simulink model "Exp2_ControlSystemDemo"  (R2017b)
settings: Solver=ode4  StartTime=0.0  StopTime=2000  FixedStep=0.001  RelTol=1e-3
InitFcn:
  | Init_control;
values from neighbouring files (symbols this model uses):
  KiPitchAttitude = 0.0552303199591522 / kFactor    (= 0.0460252666326)    [Init_control.m]
  KiPitchRate = 0.460338699849681 / kFactor    (= 0.383615583208)    [Init_control.m]
  KiRollAttitude = 0.0552303199591522 / kFactor    (= 0.0460252666326)    [Init_control.m]
  KiRollRate = 0.460338699849681 / kFactor    (= 0.383615583208)    [Init_control.m]
  KiYawRate = 0.460338699849681 / kFactor    (= 0.383615583208)    [Init_control.m]
  KpPitchAttitude = 0.630138625117681 / kFactor    (= 0.525115520931)    [Init_control.m]
  KpPitchRate = 1.31533836563383 / kFactor    (= 1.09611530469)    [Init_control.m]
  KpRollAttitude = 0.630138625117681 / kFactor    (= 0.525115520931)    [Init_control.m]
  KpRollRate = 1.31533836563383 / kFactor    (= 1.09611530469)    [Init_control.m]
  KpYawRate = 1.31533836563383 / kFactor    (= 1.09611530469)    [Init_control.m]
undefined symbols (not defined in the file or in its folder): earthRadius, ModelInit_RPM, ModelParam_envAltitude, ModelParam_GlobalNoiseGainSwitch, ModelParam_GPSLatLong, ModelParam_motorCr, ModelParam_motorJm, ModelParam_motorMinThr, ModelParam_motorT, ModelParam_motorWb, ModelParam_rotorCm, ModelParam_rotorCt, ModelParam_uavCCm, ModelParam_uavCd, ModelParam_uavDearo, ModelParam_uavJ, ModelParam_uavMass, ModelParam_uavR, ModelParam_uavType, Receive, Send
libraries: simulink x6, aerolibfltsims x4, aerolib6dof2 x1, aerolibanimutils x1
(part 1 of 2)
settings Model: SimulationMode=accelerator  Creator=dream  LastModifiedBy=dream
settings DebuggingCC: BusObjectLabelMismatch=error
settings CodeAppCC: StateflowObjectComments=on

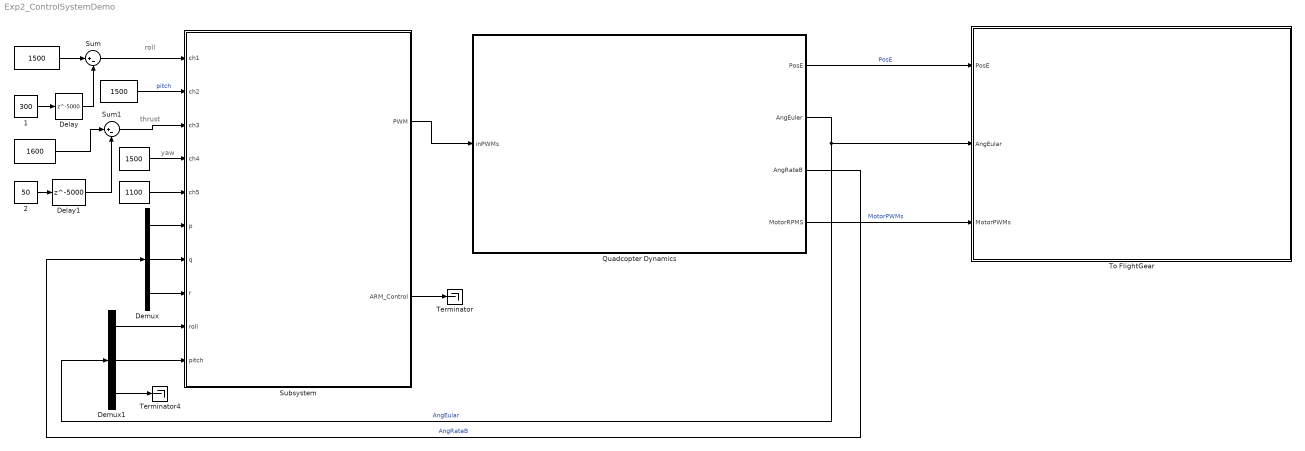
== system Exp2_ControlSystemDemo ==
  note: thrust
  note: yaw
  note: roll
  " " : Constant  Value=1100  OutDataTypeStr=uint16
  "  " : Constant  Value=1500  OutDataTypeStr=uint16
  "   " : Constant  Value=1500  OutDataTypeStr=uint16
  "      " : Constant  Value=1600  OutDataTypeStr=uint16
  "          " : Constant  Value=1500  OutDataTypeStr=uint16
  "  1" : Constant  Value=300  OutDataTypeStr=uint16
  "  2" : Constant  Value=50  OutDataTypeStr=uint16
  Delay : Delay  DelayLength=5000  InitialCondition=0
  Delay1 : Delay  DelayLength=5000  InitialCondition=0
  Demux : Demux  Outputs=3
  Demux1 : Demux  Outputs=3
  Quadcopter Dynamics : Subsystem
      mask Display: image('./icon/F450.png');
  Subsystem : Subsystem
      mask Display: image('./icon/pixhawk.png');
  Sum : Sum  Inputs=|+-
  Sum1 : Sum  Inputs=|+-
  Terminator : Terminator
  Terminator4 : Terminator
  To FlightGear : Subsystem
      mask Display: image('./icon/FlightGear.png');
  wires:
  Quadcopter Dynamics/1(PosE) -> To FlightGear/1(PosE)  "PosE"
  Quadcopter Dynamics/2(AngEuler) -> Demux1/1, To FlightGear/2(AngEular)  "AngEular"
  "   "/1 -> Subsystem/2(ch2)  "pitch"
  "          "/1 -> Subsystem/4(ch4)
  "      "/1 -> Sum1/1
  Quadcopter Dynamics/3(AngRateB) -> Demux/1  "AngRateB"
  " "/1 -> Subsystem/5(ch5)
  Demux/1 -> Subsystem/6(p)
  Demux/2 -> Subsystem/7(q)
  Demux/3 -> Subsystem/8(r)
  Demux1/1 -> Subsystem/9(roll)
  Demux1/2 -> Subsystem/10(pitch)
  Demux1/3 -> Terminator4/1
  "  "/1 -> Sum/1
  Sum/1 -> Subsystem/1(ch1)
  "  1"/1 -> Delay/1
  Delay/1 -> Sum/2
  Quadcopter Dynamics/4(MotorRPMS) -> To FlightGear/3(MotorPWMs)  "MotorPWMs"
  Sum1/1 -> Subsystem/3(ch3)
  "  2"/1 -> Delay1/1
  Delay1/1 -> Sum1/2
  Subsystem/1(PWM) -> Quadcopter Dynamics/1(inPWMs)
  Subsystem/2(ARM_Control) -> Terminator/1

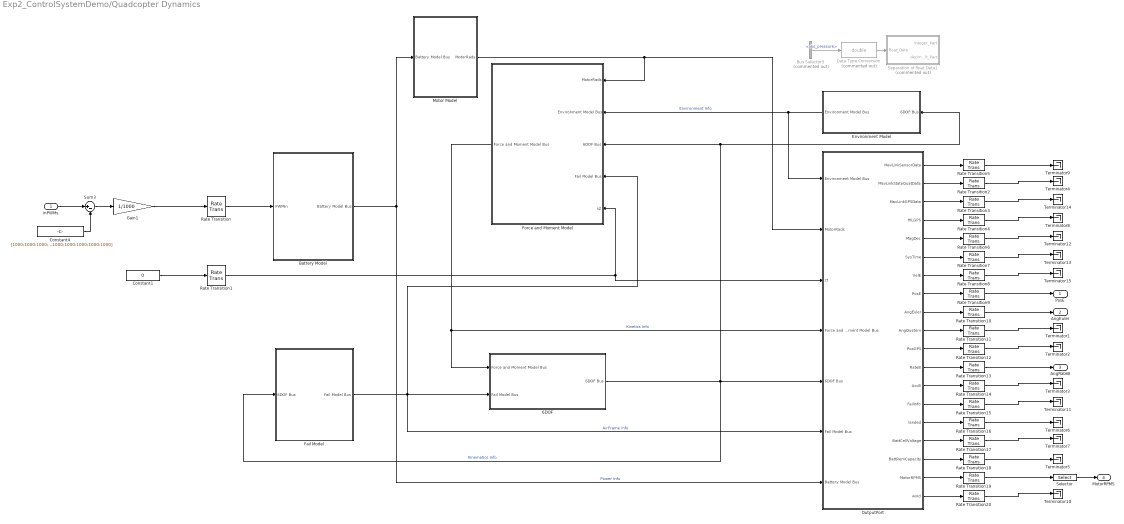
== system Exp2_ControlSystemDemo/Quadcopter Dynamics ==
  inPWMs : Inport  PortDimensions=8
  6DOF : Subsystem
  Battery Model : Subsystem
      mask help: Simulink:masks:GenSFuncDesc_MD
      mask Help: eval('feval(''rtwprivate'',''rtwhelpview'',''rtw_sfcn_block'')');
  Bus Selector3 : BusSelector  Commented=on  OutputSignals=abs_pressure
  Constant1 : Constant  Value=0
  Constant4 : Constant  Value=[1000;1000;1000;1000;1000;1000;1000;1000]
  Data Type Conversion : DataTypeConversion  Commented=on  OutDataTypeStr=double
  Environment Model : Subsystem  mask{sfcnParam1=ModelParam_GPSLatLong, sfcnParam2=ModelParam_GlobalNoiseGainSwitch, sfcnParam3=ModelParam_envAltitude}
      mask prompts: sfcnParam1 "ModelParam_GPSLatLong:"; sfcnParam2 "ModelParam_GlobalNoiseGainSwitch:"; sfcnParam3 "ModelParam_envAltitude:"
      mask help: Simulink:masks:GenSFuncDesc_MD
      mask Help: eval('feval(''rtwprivate'',''rtwhelpview'',''rtw_sfcn_block'')');
  Fail Model : Subsystem  mask{sfcnParam1=ModelParam_uavJ, sfcnParam2=ModelParam_uavMass, sfcnParam3=ModelParam_uavR}
      mask prompts: sfcnParam1 "ModelParam_uavJ:"; sfcnParam2 "ModelParam_uavMass:"; sfcnParam3 "ModelParam_uavR:"
      mask help: Simulink:masks:GenSFuncDesc_MD
      mask Help: eval('feval(''rtwprivate'',''rtwhelpview'',''rtw_sfcn_block'')');
  Force and Moment Model : Subsystem  mask{sfcnParam1=ModelParam_motorJm, sfcnParam2=ModelParam_rotorCm, sfcnParam3=ModelParam_rotorCt, sfcnParam4=ModelParam_uavCCm, sfcnParam5=ModelParam_uavCd, sfcnParam6=ModelParam_uavDearo, sfcnParam7=ModelParam_uavR, sfcnParam8=ModelParam_uavType}
      mask prompts: sfcnParam1 "ModelParam_motorJm:"; sfcnParam2 "ModelParam_rotorCm:"; sfcnParam3 "ModelParam_rotorCt:"; sfcnParam4 "ModelParam_uavCCm:"; sfcnParam5 "ModelParam_uavCd:"; sfcnParam6 "ModelParam_uavDearo:"; sfcnParam7 "ModelParam_uavR:"; sfcnParam8 "ModelParam_uavType:"
      mask help: Simulink:masks:GenSFuncDesc_MD
      mask Help: eval('feval(''rtwprivate'',''rtwhelpview'',''rtw_sfcn_block'')');
  Gain1 : Gain  Gain=1/1000
  Motor Model : Subsystem  mask{sfcnParam1=ModelInit_RPM, sfcnParam2=ModelParam_motorCr, sfcnParam3=ModelParam_motorMinThr, sfcnParam4=ModelParam_motorT, sfcnParam5=ModelParam_motorWb}
      mask prompts: sfcnParam1 "ModelInit_RPM:"; sfcnParam2 "ModelParam_motorCr:"; sfcnParam3 "ModelParam_motorMinThr:"; sfcnParam4 "ModelParam_motorT:"; sfcnParam5 "ModelParam_motorWb:"
      mask help: Simulink:masks:GenSFuncDesc_MD
      mask Help: eval('feval(''rtwprivate'',''rtwhelpview'',''rtw_sfcn_block'')');
  OutputPort : Subsystem  mask{sfcnParam1=ModelParam_GPSLatLong, sfcnParam2=ModelParam_GlobalNoiseGainSwitch, sfcnParam3=ModelParam_envAltitude}
      mask prompts: sfcnParam1 "ModelParam_GPSLatLong:"; sfcnParam2 "ModelParam_GlobalNoiseGainSwitch:"; sfcnParam3 "ModelParam_envAltitude:"
      mask help: Simulink:masks:GenSFuncDesc_MD
      mask Help: eval('feval(''rtwprivate'',''rtwhelpview'',''rtw_sfcn_block'')');
  Rate Transition{,1..20} (21 alike) : RateTransition  OutPortSampleTime=ModelParam_BusSampleRate
  Selector : Selector  InputPortWidth=8  IndexOptions=Index vector (dialog)  Indices=[1 2 3 4]  OutputSizes=1
  Separation of float Data1 : Subsystem  Commented=on  mask{IntUint=1}
      mask prompts: IntUint "整数单位"
      mask help: 分离浮点数的整数和小数部分，这样在Labview MIT模块中可以稳定输出精度
  Sum3 : Sum  Inputs=|+-
  Terminator{1..15} (15 alike) : Terminator
  PosE : Outport
  AngEuler : Outport  Port=2
  AngRateB : Outport  Port=3
  MotorRPMS : Outport  Port=4
  wires:
  Selector/1 -> MotorRPMS/1
  Constant4/1 -> Sum3/2
  inPWMs/1 -> Sum3/1
  Constant1/1 -> Rate Transition1/1
  Sum3/1 -> Gain1/1
  Rate Transition5/1 -> Terminator9/1
  Rate Transition2/1 -> Terminator4/1
  Rate Transition3/1 -> Terminator14/1
  Rate Transition4/1 -> Terminator8/1
  Rate Transition6/1 -> Terminator12/1
  Rate Transition7/1 -> Terminator13/1
  Rate Transition8/1 -> Terminator15/1
  Rate Transition9/1 -> PosE/1
  Rate Transition10/1 -> AngEuler/1
  Rate Transition11/1 -> Terminator1/1
  Rate Transition12/1 -> Terminator2/1
  Rate Transition13/1 -> AngRateB/1
  Rate Transition14/1 -> Terminator3/1
  Rate Transition15/1 -> Terminator11/1
  Rate Transition16/1 -> Terminator6/1
  Rate Transition17/1 -> Terminator7/1
  Rate Transition18/1 -> Terminator5/1
  Rate Transition19/1 -> Selector/1
  Rate Transition20/1 -> Terminator10/1
  Gain1/1 -> Rate Transition/1
  OutputPort/2(MavLinkStateQuatData) -> Rate Transition2/1
  Motor Model/1(MotorRads) -> OutputPort/2(MotorRads), Force and Moment Model/1(MotorRads)
  OutputPort/15(landed) -> Rate Transition16/1
  OutputPort/3(MavLinkGPSData) -> Rate Transition3/1
  Bus Selector3/1 -> Data Type Conversion/1  "<abs_pressure>"
  Data Type Conversion/1 -> Separation of float Data1/1(float_Data)
  OutputPort/1(MavLinkSensorData) -> Rate Transition5/1
  OutputPort/14(FailInfo) -> Rate Transition15/1
  OutputPort/13(AccB) -> Rate Transition14/1
  OutputPort/12(RateB) -> Rate Transition13/1
  OutputPort/11(PosGPS) -> Rate Transition12/1
  OutputPort/10(AngQuatern) -> Rate Transition11/1
  OutputPort/9(AngEuler) -> Rate Transition10/1
  OutputPort/8(PosE) -> Rate Transition9/1
  OutputPort/7(VelE) -> Rate Transition8/1
  OutputPort/6(SysTime) -> Rate Transition7/1
  OutputPort/5(MagDec) -> Rate Transition6/1
  OutputPort/4(HILGPS) -> Rate Transition4/1
  Battery Model/1(Battery Model Bus) -> OutputPort/7(Battery Model Bus), Motor Model/1(Battery Model Bus)  "Power Info"
  Fail Model/1(Fail Model Bus) -> OutputPort/6(Fail Model Bus), Force and Moment Model/4(Fail Model Bus), 6DOF/2(Fail Model Bus)  "AirFrame Info"
  Force and Moment Model/1(Force and Moment Model Bus) -> OutputPort/4(Force and Moment Model Bus), 6DOF/1(Force and Moment Model Bus)  "Kinetics Info"
  6DOF/1(6DOF Bus) -> OutputPort/5(6DOF Bus), Fail Model/1(6DOF Bus), Environment Model/1(6DOF Bus), Force and Moment Model/3(6DOF Bus)  "Kinematics Info"
  Environment Model/1(Environment Model Bus) -> OutputPort/1(Environment Model Bus), Force and Moment Model/2(Environment Model Bus)  "Environment Info"
  OutputPort/16(BattCellVoltage) -> Rate Transition17/1
  OutputPort/17(BattRemCapacity) -> Rate Transition18/1
  OutputPort/19(wind) -> Rate Transition20/1
  OutputPort/18(MotorRPMS) -> Rate Transition19/1
  Rate Transition/1 -> Battery Model/1(PWMin)
  Rate Transition1/1 -> OutputPort/3(zt), Force and Moment Model/5("tZ ")

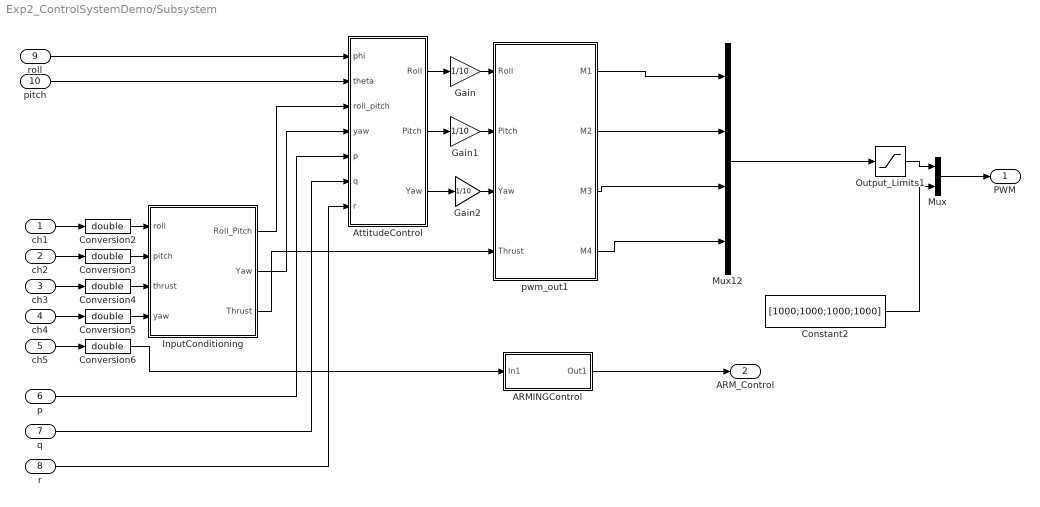
== system Exp2_ControlSystemDemo/Subsystem ==
  ch1 : Inport  OutDataTypeStr=uint16  PortDimensions=1
  ch2 : Inport  Port=2  OutDataTypeStr=uint16  PortDimensions=1
  ch3 : Inport  Port=3  OutDataTypeStr=uint16  PortDimensions=1
  ch4 : Inport  Port=4  OutDataTypeStr=uint16  PortDimensions=1
  ch5 : Inport  Port=5  OutDataTypeStr=uint16  PortDimensions=1  Interpolate=off
  p : Inport  Port=6  PortDimensions=1
  q : Inport  Port=7  PortDimensions=1
  r : Inport  Port=8  PortDimensions=1
  roll : Inport  Port=9  PortDimensions=1
  pitch : Inport  Port=10  PortDimensions=1
  ARMINGControl : Subsystem
  AttitudeControl : Subsystem
  Constant2 : Constant  Value=[1000;1000;1000;1000]
  Conversion{2..6} (5 alike) : DataTypeConversion  OutDataTypeStr=double
  Gain : Gain  Gain=1/10
  Gain1 : Gain  Gain=1/10
  Gain2 : Gain  Gain=1/10
  InputConditioning : Subsystem
  Mux : Mux  Inputs=2
  Mux12 : Mux
  Output_Limits1 : Saturate  UpperLimit=2000  LowerLimit=1000
  pwm_out1 : MATLAB Function  TreatAsAtomicUnit=on  SystemSampleTime=0.004
  PWM : Outport  PortDimensions=8
  ARM_Control : Outport  Port=2  PortDimensions=1
  wires:
  InputConditioning/3(Thrust) -> pwm_out1/4(Thrust)
  q/1 -> AttitudeControl/6(q)
  ARMINGControl/1(Out1) -> ARM_Control/1
  Gain1/1 -> pwm_out1/2(Pitch)
  pitch/1 -> AttitudeControl/2(theta)
  Gain/1 -> pwm_out1/1(Roll)
  Conversion5/1 -> InputConditioning/4(yaw)
  Output_Limits1/1 -> Mux/1
  pwm_out1/1(M1) -> Mux12/1
  Gain2/1 -> pwm_out1/3(Yaw)
  pwm_out1/2(M2) -> Mux12/2
  ch4/1 -> Conversion5/1
  r/1 -> AttitudeControl/7(r)
  AttitudeControl/3(Yaw) -> Gain2/1
  ch2/1 -> Conversion3/1
  ch5/1 -> Conversion6/1
  roll/1 -> AttitudeControl/1(phi)
  Conversion3/1 -> InputConditioning/2(pitch)
  Conversion4/1 -> InputConditioning/3(thrust)
  Conversion6/1 -> ARMINGControl/1(In1)
  Mux12/1 -> Output_Limits1/1
  Conversion2/1 -> InputConditioning/1(roll)
  AttitudeControl/2(Pitch) -> Gain1/1
  AttitudeControl/1(Roll) -> Gain/1
  ch1/1 -> Conversion2/1
  pwm_out1/4(M4) -> Mux12/4
  p/1 -> AttitudeControl/5(p)
  ch3/1 -> Conversion4/1
  InputConditioning/1(Roll_Pitch) -> AttitudeControl/3(roll_pitch)
  pwm_out1/3(M3) -> Mux12/3
  Constant2/1 -> Mux/2
  Mux/1 -> PWM/1
  InputConditioning/2(Yaw) -> AttitudeControl/4(yaw)

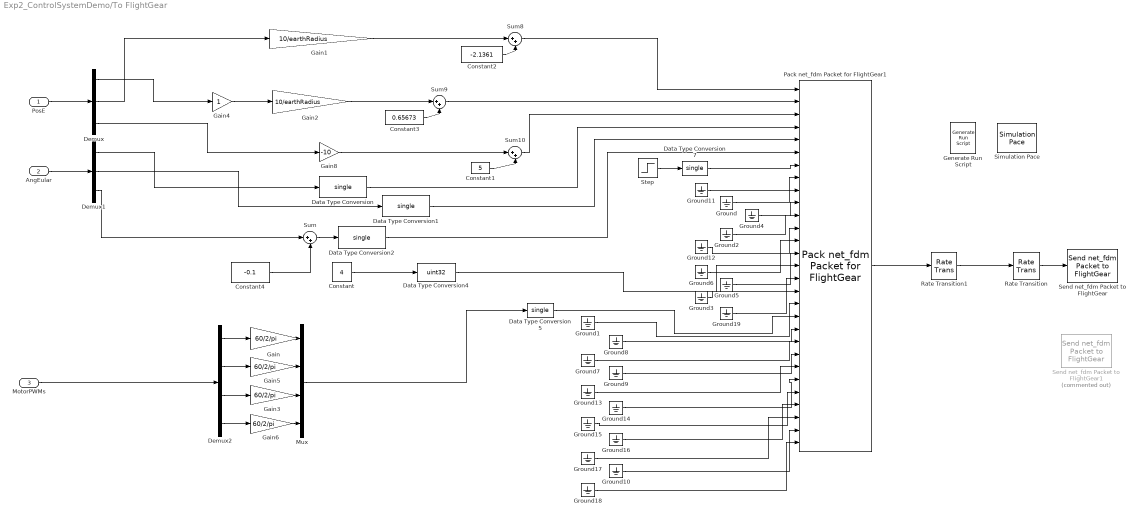
== system Exp2_ControlSystemDemo/To FlightGear ==
  PosE : Inport
  AngEular : Inport  Port=2
  MotorPWMs : Inport  Port=3
  Constant : Constant  Value=4
  Constant1 : Constant  Value=5  VectorParams1D=off
  Constant2 : Constant  Value=-2.1361  VectorParams1D=off
  Constant3 : Constant  Value=0.65673  VectorParams1D=off
  Constant4 : Constant  Value=-0.1  VectorParams1D=off
  Data Type Conversion : DataTypeConversion  OutDataTypeStr=single  SaturateOnIntegerOverflow=on
  Data Type Conversion1 : DataTypeConversion  OutDataTypeStr=single  SaturateOnIntegerOverflow=on
  Data Type Conversion2 : DataTypeConversion  OutDataTypeStr=single  SaturateOnIntegerOverflow=on
  Data Type Conversion4 : DataTypeConversion  OutDataTypeStr=uint32
  Data Type Conversion5 : DataTypeConversion  OutDataTypeStr=single
  Data Type Conversion7 : DataTypeConversion  OutDataTypeStr=single
  Demux : Demux  Outputs=3
  Demux1 : Demux  Outputs=3
  Demux2 : Demux
  Gain{,3,5..6} (4 alike) : Gain  Gain=60/2/pi
  Gain1 : Gain  Gain=10/earthRadius
  Gain2 : Gain  Gain=10/earthRadius
  Gain4 : Gain
  Gain8 : Gain  Gain=-10
  Generate Run Script : aerolibfltsims/Generate Run Script  OutputFileName=runfg.bat  FlightGearBaseDirectory=C:\Program Files\FlightGear 2016.1.2  GeometryModelName=Rotor4  DestinationPort=5502  OriginAddress=127.0.0.1  OriginPort=5505  LocalAddress=127.0.0.1  AirportId=KSF0  RunwayId=10L  InitialAltitude=0  InitialHeading=0  OffsetDistance=0  OffsetAzimuth=0  GenerateFile=off  Architecture=Default  dataFlow=Send-Receive
  Ground{,1..19} (20 alike) : Ground
  Mux : Mux
  Pack net_fdm Packet for FlightGear1 : aerolibfltsims/Pack net_fdm Packet for FlightGear  FlightGearVersion=v2016.1  ShowPositionAttitudeInputs=on  ShowVelocityAccelerationInputs=off  ShowControlSurfacePositionInputs=on  ShowEngineFuelInputs=on  ShowLandingGearInputs=off  ShowEnvironmentInputs=off  SampleTime=0.01
      settings: SourceProductName=Aerospace Blockset  SourceProductBaseCode=AE
  Rate Transition : RateTransition
  Rate Transition1 : RateTransition
  Send net_fdm Packet to FlightGear : aerolibfltsims/Send net_fdm Packet to FlightGear  DestinationIpAddress=127.0.0.1  DestinationPort=5502  LocalIpPort=-1  varLen=off  SampleTime=0.005
      settings: SourceProductName=Aerospace Blockset  SourceProductBaseCode=AE
  Send net_fdm Packet to FlightGear1 : aerolibfltsims/Send net_fdm Packet to FlightGear  Commented=on  DestinationIpAddress=192.168.199.46  DestinationPort=5502  LocalIpPort=-1  varLen=off  SampleTime=0.01
      settings: SourceProductName=Aerospace Blockset  SourceProductBaseCode=AE
  Simulation Pace : aerolibanimutils/Simulation Pace  SimulationPace=1  SleepMode=MATLAB Thread  OutputPaceError=off  SampleTime=-1
      settings: AttributesFormatString=%<SimulationPace> sec/sec
  Step : Step  Time=5  SampleTime=0
  Sum{,8..10} (4 alike) : Sum  Inputs=|++
  wires:
  Rate Transition/1 -> Send net_fdm Packet to FlightGear/1
  Demux/1 -> Gain4/1
  Demux/2 -> Gain1/1
  Demux/3 -> Gain8/1
  Constant4/1 -> Sum/2
  Sum/1 -> Data Type Conversion2/1
  Gain1/1 -> Sum8/1
  Constant2/1 -> Sum8/2
  Gain2/1 -> Sum9/1
  Constant3/1 -> Sum9/2
  Constant1/1 -> Sum10/2
  Gain8/1 -> Sum10/1
  Pack net_fdm Packet for FlightGear1/1 -> Rate Transition1/1
  Demux1/2 -> Data Type Conversion1/1
  Demux1/3 -> Sum/1
  Data Type Conversion7/1 -> Pack net_fdm Packet for FlightGear1/7
  Ground8/1 -> Pack net_fdm Packet for FlightGear1/20
  Ground/1 -> Pack net_fdm Packet for FlightGear1/9
  Ground7/1 -> Pack net_fdm Packet for FlightGear1/21
  Ground9/1 -> Pack net_fdm Packet for FlightGear1/22
  Ground13/1 -> Pack net_fdm Packet for FlightGear1/23
  Ground14/1 -> Pack net_fdm Packet for FlightGear1/24
  Ground15/1 -> Pack net_fdm Packet for FlightGear1/25
  Ground16/1 -> Pack net_fdm Packet for FlightGear1/26
  Ground17/1 -> Pack net_fdm Packet for FlightGear1/27
  Ground10/1 -> Pack net_fdm Packet for FlightGear1/28
  Ground18/1 -> Pack net_fdm Packet for FlightGear1/29
  Step/1 -> Data Type Conversion7/1
  Data Type Conversion4/1 -> Pack net_fdm Packet for FlightGear1/17
  Ground1/1 -> Pack net_fdm Packet for FlightGear1/18
  Ground3/1 -> Pack net_fdm Packet for FlightGear1/15
  Ground5/1 -> Pack net_fdm Packet for FlightGear1/14
  Ground6/1 -> Pack net_fdm Packet for FlightGear1/13
  Ground4/1 -> Pack net_fdm Packet for FlightGear1/10
  Ground11/1 -> Pack net_fdm Packet for FlightGear1/8
  Data Type Conversion2/1 -> Pack net_fdm Packet for FlightGear1/6
  Data Type Conversion1/1 -> Pack net_fdm Packet for FlightGear1/5
  Data Type Conversion/1 -> Pack net_fdm Packet for FlightGear1/4
  Sum8/1 -> Pack net_fdm Packet for FlightGear1/1
  Sum9/1 -> Pack net_fdm Packet for FlightGear1/2
  Sum10/1 -> Pack net_fdm Packet for FlightGear1/3
  Constant/1 -> Data Type Conversion4/1
  Data Type Conversion5/1 -> Pack net_fdm Packet for FlightGear1/19
  Ground2/1 -> Pack net_fdm Packet for FlightGear1/11
  Ground12/1 -> Pack net_fdm Packet for FlightGear1/12
  Ground19/1 -> Pack net_fdm Packet for FlightGear1/16
  Gain4/1 -> Gain2/1
  AngEular/1 -> Demux1/1
  PosE/1 -> Demux/1
  MotorPWMs/1 -> Demux2/1
  Mux/1 -> Data Type Conversion5/1
  Demux2/1 -> Gain/1
  Demux2/3 -> Gain3/1
  Gain/1 -> Mux/1
  Gain3/1 -> Mux/3
  Demux2/2 -> Gain5/1
  Gain5/1 -> Mux/2
  Demux2/4 -> Gain6/1
  Gain6/1 -> Mux/4
  Demux1/1 -> Data Type Conversion/1
  Rate Transition1/1 -> Rate Transition/1

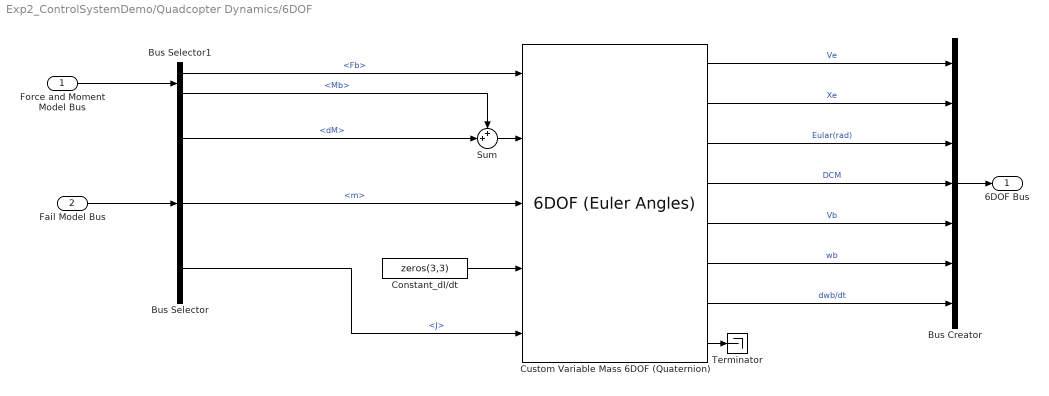
== system Exp2_ControlSystemDemo/Quadcopter Dynamics/6DOF ==
  Force and Moment Model Bus : Inport
  Fail Model Bus : Inport  Port=2
  Bus Creator : BusCreator  Inputs=7
  Bus Selector : BusSelector  OutputSignals=dM,m,J
  Bus Selector1 : BusSelector  OutputSignals=Fb,Mb
  Constant_dI/dt : Constant  Value=zeros(3,3)
  Custom Variable Mass 6DOF (Quaternion) : aerolib6dof2/6DOF (Euler Angles)  units=Metric (MKS)  mtype=Custom Variable  rep=Quaternion  xme_0=ModelInit_PosE  Vm_0=ModelInit_VelB  eul_0=ModelInit_AngEuler  pm_0=ModelInit_RateB  mass_0=1.0  mass_e=0.5  mass_f=2.0  inertia=eye(3)  inertia_e=eye(3)  inertia_f=2*eye(3)  k_quat=1.0  vre_flag=off
      settings: SourceProductName=Aerospace Blockset  SourceProductBaseCode=AE
  Sum : Sum  Inputs=++|
  Terminator : Terminator
  6DOF Bus : Outport
  wires:
  Bus Selector1/1 -> Custom Variable Mass 6DOF (Quaternion)/1  "<Fb>"
  Bus Selector/2 -> Custom Variable Mass 6DOF (Quaternion)/3  "<m>"
  Custom Variable Mass 6DOF (Quaternion)/8 -> Terminator/1
  Sum/1 -> Custom Variable Mass 6DOF (Quaternion)/2
  Constant_dI/dt/1 -> Custom Variable Mass 6DOF (Quaternion)/4
  Custom Variable Mass 6DOF (Quaternion)/5 -> Bus Creator/5  "Vb"
  Custom Variable Mass 6DOF (Quaternion)/6 -> Bus Creator/6  "wb"
  Custom Variable Mass 6DOF (Quaternion)/1 -> Bus Creator/1  "Ve"
  Custom Variable Mass 6DOF (Quaternion)/4 -> Bus Creator/4  "DCM"
  Custom Variable Mass 6DOF (Quaternion)/2 -> Bus Creator/2  "Xe"
  Custom Variable Mass 6DOF (Quaternion)/3 -> Bus Creator/3  "Eular(rad)"
  Custom Variable Mass 6DOF (Quaternion)/7 -> Bus Creator/7  "dwb/dt"
  Bus Selector/3 -> Custom Variable Mass 6DOF (Quaternion)/5  "<J>"
  Bus Selector/1 -> Sum/2  "<dM>"
  Bus Selector1/2 -> Sum/1  "<Mb>"
  Fail Model Bus/1 -> Bus Selector/1
  Force and Moment Model Bus/1 -> Bus Selector1/1
  Bus Creator/1 -> 6DOF Bus/1

== system Exp2_ControlSystemDemo/Quadcopter Dynamics/Battery Model ==
  PWMin : Inport
  Battery Model_sfcn : S-Function  FunctionName=Battery_sf  SFunctionModules=""  SFunctionDeploymentMode=off  EnableBusSupport=off  mask{rtw_sf_name=Battery_sf, showVar=off}
      mask prompts: rtw_sf_name "Simulink:masks:GenSFuncName_MP"; showVar "Simulink:masks:GenSFuncShowModuleList_MP"
      mask help: Simulink:masks:GenSFuncDesc_MD
      mask init:
      | displist = '';
      | if ~strcmp(get_param(gcb, 'FunctionName'), rtw_sf_name);
      |   set_param(gcb, 'FunctionName', rtw_sf_name);
      | end
      | % Check if we are generating code
      | rtw_mode = false;
      | if strcmpi(get_param(bdroot(gcb),'SimulationStatus'),'Initializing')
      | 	rtw_mode = strcmpi(get_param(bdroot(gcb),'BuildingRTWCode'),'on') && ...
      | 		~strcmpi(get_param(bdroot(gcb),'TargetStyle'),'SimulationTarget');
      | end
      | if showVar || rtw_mode
      | 	if exist('rtwsfunc') == 2 | exist('rtwsfunc') == 6
      | 		tmplist = rtwsfunc(rtw_sf_name,gcb);
      | 		tmplist = DAStudio.message('Simulink:masks:GenSFuncListOfModules_IC', tmplist);
      | 	elseif showVar
      | 		tmplist1 = DAStudio.message('Simulink:masks:GenSFuncListOfModules_IC', '');
      |         tmplist2 = DAStudio.message('Simulink:masks:GenSFuncNotLicensed_IC');
      |         tmplist = [tmplist1 tmplist2];
      |  	end
      | end
      | if showVar
      |   displist = tmplist;
      | end
      settings: CopyFcn=|
      | if ~strcmp(get_param(gcb,'Linkstatus'),'none') && ...
      | ~strcmp(get_param(gcb,'Linkstatus'),'implicit')
      |   set_param(gcb,'LinkStatus','none');
      | end
      mask Help: eval('feval(''rtwprivate'',''rtwhelpview'',''rtw_sfcn_block'')');
      mask Display:
      | port_label('input',1,'PWMin');
      | port_label('output',1,'PWMOut');
      | port_label('output',2,'cellVol');
      | port_label('output',3,'remCapa');
  __InputSSForSFun__ : Subsystem
  __OutputSSForSFun__ : Subsystem
  Battery Model Bus : Outport
  wires:
  PWMin/1 -> __InputSSForSFun__/1(PWMin)
  __InputSSForSFun__/1(__UniqueOutportName__1__) -> Battery Model_sfcn/1
  Battery Model_sfcn/1 -> __OutputSSForSFun__/1(__UniqueInportName__1__)
  Battery Model_sfcn/2 -> __OutputSSForSFun__/2(__UniqueInportName__2__)
  Battery Model_sfcn/3 -> __OutputSSForSFun__/3(__UniqueInportName__3__)
  __OutputSSForSFun__/1(Battery Model Bus) -> Battery Model Bus/1

== system Exp2_ControlSystemDemo/Quadcopter Dynamics/Environment Model ==
  6DOF Bus : Inport
  Environment Model_sfcn : S-Function  FunctionName=Environment_sf  Parameters=sfcnParam1, sfcnParam2, sfcnParam3  SFunctionModules=""  SFunctionDeploymentMode=off  EnableBusSupport=off  SFcnStateName=DWORK0  mask{rtw_sf_name=Environment_sf, showVar=off, sfcnParam1=sfcnParam1, sfcnParam2=sfcnParam2, sfcnParam3=sfcnParam3}
      mask prompts: rtw_sf_name "Simulink:masks:GenSFuncName_MP"; showVar "Simulink:masks:GenSFuncShowModuleList_MP"; sfcnParam1 "ModelParam_GPSLatLong:"; sfcnParam2 "ModelParam_GlobalNoiseGainSwitch:"; sfcnParam3 "ModelParam_envAltitude:"
      mask help: Simulink:masks:GenSFuncDesc_MD
      mask init: same as Exp2_ControlSystemDemo/Quadcopter Dynamics/Battery Model/Battery Model_sfcn
      settings: SFcnIsStateOwnerBlock=on
      settings: CopyFcn=|
      | if ~strcmp(get_param(gcb,'Linkstatus'),'none') && ...
      | ~strcmp(get_param(gcb,'Linkstatus'),'implicit')
      |   set_param(gcb,'LinkStatus','none');
      | end
      mask Help: eval('feval(''rtwprivate'',''rtwhelpview'',''rtw_sfcn_block'')');
      mask Display:
      | port_label('input',1,'Ve');
      | port_label('input',2,'Xe');
      | port_label('input',3,'Eular(rad)');
      | port_label('input',4,'DCM');
      | port_label('input',5,'Vb');
      | port_label('input',6,'wb');
      | port_label('input',7,'dwb/dt');
      | port_label('output',1,'PosGPS');
      | port_label('output',2,'gravity');
      | port_label('output',3,'TempC');
      | port_label('output',4,'AirPressure');
      | port_label('output',5,'Rho');
      | port_label('output',6,'Windb');
      | port_label('output',7,'Wind');
  __InputSSForSFun__ : Subsystem
  __OutputSSForSFun__ : Subsystem
  Environment Model Bus : Outport
  wires:
  6DOF Bus/1 -> __InputSSForSFun__/1(6DOF Bus)
  __InputSSForSFun__/1(__UniqueOutportName__1__) -> Environment Model_sfcn/1
  __InputSSForSFun__/2(__UniqueOutportName__2__) -> Environment Model_sfcn/2
  __InputSSForSFun__/3(__UniqueOutportName__3__) -> Environment Model_sfcn/3
  __InputSSForSFun__/4(__UniqueOutportName__4__) -> Environment Model_sfcn/4
  __InputSSForSFun__/5(__UniqueOutportName__5__) -> Environment Model_sfcn/5
  __InputSSForSFun__/6(__UniqueOutportName__6__) -> Environment Model_sfcn/6
  __InputSSForSFun__/7(__UniqueOutportName__7__) -> Environment Model_sfcn/7
  Environment Model_sfcn/1 -> __OutputSSForSFun__/1(__UniqueInportName__1__)
  Environment Model_sfcn/2 -> __OutputSSForSFun__/2(__UniqueInportName__2__)
  Environment Model_sfcn/3 -> __OutputSSForSFun__/3(__UniqueInportName__3__)
  Environment Model_sfcn/4 -> __OutputSSForSFun__/4(__UniqueInportName__4__)
  Environment Model_sfcn/5 -> __OutputSSForSFun__/5(__UniqueInportName__5__)
  Environment Model_sfcn/6 -> __OutputSSForSFun__/6(__UniqueInportName__6__)
  Environment Model_sfcn/7 -> __OutputSSForSFun__/7(__UniqueInportName__7__)
  __OutputSSForSFun__/1(Environment Model Bus) -> Environment Model Bus/1

== system Exp2_ControlSystemDemo/Quadcopter Dynamics/Fail Model ==
  6DOF Bus : Inport
  Fail Model_sfcn : S-Function  FunctionName=Fail_sf  Parameters=sfcnParam1, sfcnParam2, sfcnParam3  SFunctionModules=""  SFunctionDeploymentMode=off  EnableBusSupport=off  mask{rtw_sf_name=Fail_sf, showVar=off, sfcnParam1=sfcnParam1, sfcnParam2=sfcnParam2, sfcnParam3=sfcnParam3}
      mask prompts: rtw_sf_name "Simulink:masks:GenSFuncName_MP"; showVar "Simulink:masks:GenSFuncShowModuleList_MP"; sfcnParam1 "ModelParam_uavJ:"; sfcnParam2 "ModelParam_uavMass:"; sfcnParam3 "ModelParam_uavR:"
      mask help: Simulink:masks:GenSFuncDesc_MD
      mask init: same as Exp2_ControlSystemDemo/Quadcopter Dynamics/Battery Model/Battery Model_sfcn
      settings: CopyFcn=|
      | if ~strcmp(get_param(gcb,'Linkstatus'),'none') && ...
      | ~strcmp(get_param(gcb,'Linkstatus'),'implicit')
      |   set_param(gcb,'LinkStatus','none');
      | end
      mask Help: eval('feval(''rtwprivate'',''rtwhelpview'',''rtw_sfcn_block'')');
      mask Display:
      | port_label('input',1,'Ve');
      | port_label('input',2,'Xe');
      | port_label('input',3,'Eular(rad)');
      | port_label('input',4,'DCM');
      | port_label('input',5,'Vb');
      | port_label('input',6,'wb');
      | port_label('input',7,'dwb/dt');
      | port_label('output',1,'m');
      | port_label('output',2,'J');
      | port_label('output',3,'dM');
  __InputSSForSFun__ : Subsystem
  __OutputSSForSFun__ : Subsystem
  Fail Model Bus : Outport
  wires:
  6DOF Bus/1 -> __InputSSForSFun__/1(6DOF Bus)
  __InputSSForSFun__/1(__UniqueOutportName__1__) -> Fail Model_sfcn/1
  __InputSSForSFun__/2(__UniqueOutportName__2__) -> Fail Model_sfcn/2
  __InputSSForSFun__/3(__UniqueOutportName__3__) -> Fail Model_sfcn/3
  __InputSSForSFun__/4(__UniqueOutportName__4__) -> Fail Model_sfcn/4
  __InputSSForSFun__/5(__UniqueOutportName__5__) -> Fail Model_sfcn/5
  __InputSSForSFun__/6(__UniqueOutportName__6__) -> Fail Model_sfcn/6
  __InputSSForSFun__/7(__UniqueOutportName__7__) -> Fail Model_sfcn/7
  Fail Model_sfcn/1 -> __OutputSSForSFun__/1(__UniqueInportName__1__)
  Fail Model_sfcn/2 -> __OutputSSForSFun__/2(__UniqueInportName__2__)
  Fail Model_sfcn/3 -> __OutputSSForSFun__/3(__UniqueInportName__3__)
  __OutputSSForSFun__/1(Fail Model Bus) -> Fail Model Bus/1

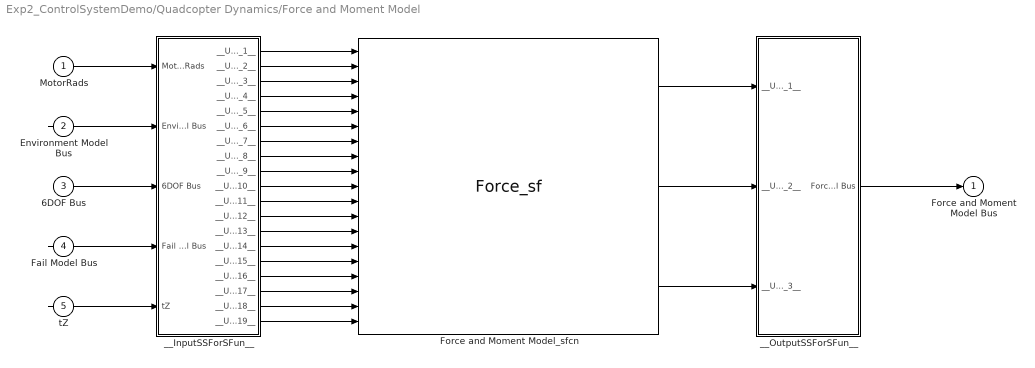
== system Exp2_ControlSystemDemo/Quadcopter Dynamics/Force and Moment Model ==
  MotorRads : Inport
  Environment Model Bus : Inport  Port=2
  6DOF Bus : Inport  Port=3
  Fail Model Bus : Inport  Port=4
  "tZ " : Inport  Port=5
  Force and Moment Model_sfcn : S-Function  FunctionName=Force_sf  Parameters=sfcnParam1, sfcnParam2, sfcnParam3, sfcnParam4, sfcnParam5, sfcnParam6, sfcnParam7, sfcnParam8  SFunctionModules=""  SFunctionDeploymentMode=off  EnableBusSupport=off  mask{rtw_sf_name=Force_sf, showVar=off, sfcnParam1=sfcnParam1, sfcnParam2=sfcnParam2, sfcnParam3=sfcnParam3, sfcnParam4=sfcnParam4, sfcnParam5=sfcnParam5, sfcnParam6=sfcnParam6, sfcnParam7=sfcnParam7, sfcnParam8=sfcnParam8}
      mask prompts: rtw_sf_name "Simulink:masks:GenSFuncName_MP"; showVar "Simulink:masks:GenSFuncShowModuleList_MP"; sfcnParam1 "ModelParam_motorJm:"; sfcnParam2 "ModelParam_rotorCm:"; sfcnParam3 "ModelParam_rotorCt:"; sfcnParam4 "ModelParam_uavCCm:"; sfcnParam5 "ModelParam_uavCd:"; sfcnParam6 "ModelParam_uavDearo:"; sfcnParam7 "ModelParam_uavR:"; sfcnParam8 "ModelParam_uavType:"
      mask help: Simulink:masks:GenSFuncDesc_MD
      mask init: same as Exp2_ControlSystemDemo/Quadcopter Dynamics/Battery Model/Battery Model_sfcn
      settings: CopyFcn=|
      | if ~strcmp(get_param(gcb,'Linkstatus'),'none') && ...
      | ~strcmp(get_param(gcb,'Linkstatus'),'implicit')
      |   set_param(gcb,'LinkStatus','none');
      | end
      mask Help: eval('feval(''rtwprivate'',''rtwhelpview'',''rtw_sfcn_block'')');
      mask Display:
      | port_label('input',1,'MotorRads');
      | port_label('input',2,'PosGPS');
      | port_label('input',3,'gravity');
      | port_label('input',4,'TempC');
      | port_label('input',5,'AirPressure');
      | port_label('input',6,'Rho');
      | port_label('input',7,'Windb');
      | port_label('input',8,'Wind');
      | port_label('input',9,'Ve');
      | port_label('input',10,'Xe');
      | port_label('input',11,'Eular(rad)');
      | port_label('input',12,'DCM');
      | port_label('input',13,'Vb');
      | port_label('input',14,'wb');
      | port_label('input',15,'dwb/dt');
      | port_label('input',16,'m');
      | port_label('input',17,'J');
      | port_label('input',18,'dM');
      | port_label('input',19,'tZ ');
      | port_label('output',1,'Fb');
      | port_label('output',2,'Mb');
      | port_label('output',3,'landed');
  __InputSSForSFun__ : Subsystem
  __OutputSSForSFun__ : Subsystem
  Force and Moment Model Bus : Outport
  wires:
  MotorRads/1 -> __InputSSForSFun__/1(MotorRads)
  Environment Model Bus/1 -> __InputSSForSFun__/2(Environment Model Bus)
  6DOF Bus/1 -> __InputSSForSFun__/3(6DOF Bus)
  Fail Model Bus/1 -> __InputSSForSFun__/4(Fail Model Bus)
  "tZ "/1 -> __InputSSForSFun__/5("tZ ")
  __InputSSForSFun__/1(__UniqueOutportName__1__) -> Force and Moment Model_sfcn/1
  __InputSSForSFun__/2(__UniqueOutportName__2__) -> Force and Moment Model_sfcn/2
  __InputSSForSFun__/3(__UniqueOutportName__3__) -> Force and Moment Model_sfcn/3
  __InputSSForSFun__/4(__UniqueOutportName__4__) -> Force and Moment Model_sfcn/4
  __InputSSForSFun__/5(__UniqueOutportName__5__) -> Force and Moment Model_sfcn/5
  __InputSSForSFun__/6(__UniqueOutportName__6__) -> Force and Moment Model_sfcn/6
  __InputSSForSFun__/7(__UniqueOutportName__7__) -> Force and Moment Model_sfcn/7
  __InputSSForSFun__/8(__UniqueOutportName__8__) -> Force and Moment Model_sfcn/8
  __InputSSForSFun__/9(__UniqueOutportName__9__) -> Force and Moment Model_sfcn/9
  __InputSSForSFun__/10(__UniqueOutportName__10__) -> Force and Moment Model_sfcn/10
  __InputSSForSFun__/11(__UniqueOutportName__11__) -> Force and Moment Model_sfcn/11
  __InputSSForSFun__/12(__UniqueOutportName__12__) -> Force and Moment Model_sfcn/12
  __InputSSForSFun__/13(__UniqueOutportName__13__) -> Force and Moment Model_sfcn/13
  __InputSSForSFun__/14(__UniqueOutportName__14__) -> Force and Moment Model_sfcn/14
  __InputSSForSFun__/15(__UniqueOutportName__15__) -> Force and Moment Model_sfcn/15
  __InputSSForSFun__/16(__UniqueOutportName__16__) -> Force and Moment Model_sfcn/16
  __InputSSForSFun__/17(__UniqueOutportName__17__) -> Force and Moment Model_sfcn/17
  __InputSSForSFun__/18(__UniqueOutportName__18__) -> Force and Moment Model_sfcn/18
  __InputSSForSFun__/19(__UniqueOutportName__19__) -> Force and Moment Model_sfcn/19
  Force and Moment Model_sfcn/1 -> __OutputSSForSFun__/1(__UniqueInportName__1__)
  Force and Moment Model_sfcn/2 -> __OutputSSForSFun__/2(__UniqueInportName__2__)
  Force and Moment Model_sfcn/3 -> __OutputSSForSFun__/3(__UniqueInportName__3__)
  __OutputSSForSFun__/1(Force and Moment Model Bus) -> Force and Moment Model Bus/1

== system Exp2_ControlSystemDemo/Quadcopter Dynamics/Motor Model ==
  Battery Model Bus : Inport
  Motor Model_sfcn : S-Function  FunctionName=Motor_sf  Parameters=sfcnParam1, sfcnParam2, sfcnParam3, sfcnParam4, sfcnParam5  SFunctionModules=""  SFunctionDeploymentMode=off  EnableBusSupport=off  mask{rtw_sf_name=Motor_sf, showVar=off, sfcnParam1=sfcnParam1, sfcnParam2=sfcnParam2, sfcnParam3=sfcnParam3, sfcnParam4=sfcnParam4, sfcnParam5=sfcnParam5}
      mask prompts: rtw_sf_name "Simulink:masks:GenSFuncName_MP"; showVar "Simulink:masks:GenSFuncShowModuleList_MP"; sfcnParam1 "ModelInit_RPM:"; sfcnParam2 "ModelParam_motorCr:"; sfcnParam3 "ModelParam_motorMinThr:"; sfcnParam4 "ModelParam_motorT:"; sfcnParam5 "ModelParam_motorWb:"
      mask help: Simulink:masks:GenSFuncDesc_MD
      mask init: same as Exp2_ControlSystemDemo/Quadcopter Dynamics/Battery Model/Battery Model_sfcn
      settings: CopyFcn=|
      | if ~strcmp(get_param(gcb,'Linkstatus'),'none') && ...
      | ~strcmp(get_param(gcb,'Linkstatus'),'implicit')
      |   set_param(gcb,'LinkStatus','none');
      | end
      mask Help: eval('feval(''rtwprivate'',''rtwhelpview'',''rtw_sfcn_block'')');
      mask Display:
      | port_label('input',1,'PWMOut');
      | port_label('input',2,'cellVol');
      | port_label('input',3,'remCapa');
      | port_label('output',1,'MotorRads');
  __InputSSForSFun__ : Subsystem
  __OutputSSForSFun__ : Subsystem
  MotorRads : Outport
  wires:
  Battery Model Bus/1 -> __InputSSForSFun__/1(Battery Model Bus)
  __InputSSForSFun__/1(__UniqueOutportName__1__) -> Motor Model_sfcn/1
  __InputSSForSFun__/2(__UniqueOutportName__2__) -> Motor Model_sfcn/2
  __InputSSForSFun__/3(__UniqueOutportName__3__) -> Motor Model_sfcn/3
  Motor Model_sfcn/1 -> __OutputSSForSFun__/1(__UniqueInportName__1__)
  __OutputSSForSFun__/1(MotorRads) -> MotorRads/1

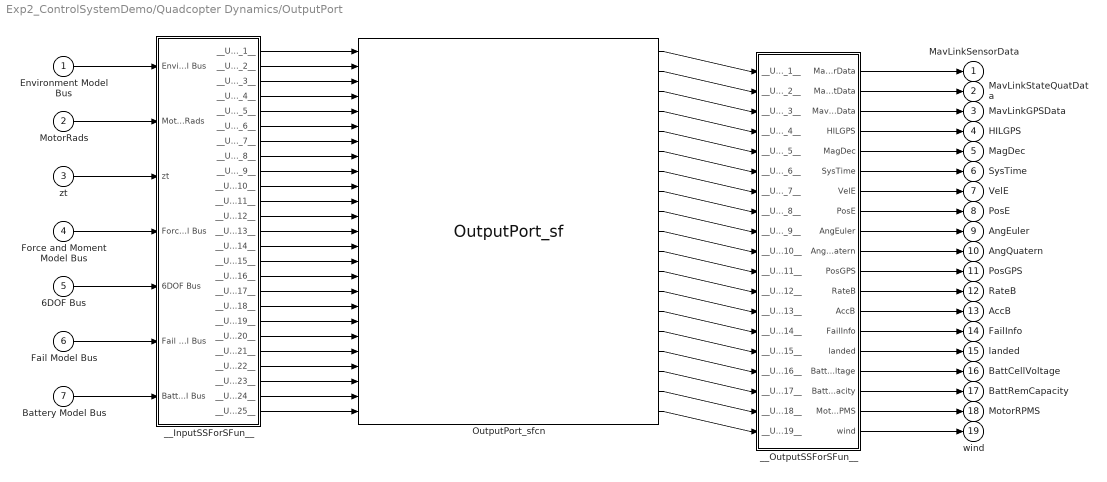
== system Exp2_ControlSystemDemo/Quadcopter Dynamics/OutputPort ==
  Environment Model Bus : Inport
  MotorRads : Inport  Port=2
  zt : Inport  Port=3
  Force and Moment Model Bus : Inport  Port=4
  6DOF Bus : Inport  Port=5
  Fail Model Bus : Inport  Port=6
  Battery Model Bus : Inport  Port=7
  OutputPort_sfcn : S-Function  FunctionName=OutputPort_sf  Parameters=sfcnParam1, sfcnParam2, sfcnParam3  SFunctionModules=""  SFunctionDeploymentMode=off  EnableBusSupport=off  SFcnStateName=DWORK0  mask{rtw_sf_name=OutputPort_sf, showVar=off, sfcnParam1=sfcnParam1, sfcnParam2=sfcnParam2, sfcnParam3=sfcnParam3}
      mask prompts: rtw_sf_name "Simulink:masks:GenSFuncName_MP"; showVar "Simulink:masks:GenSFuncShowModuleList_MP"; sfcnParam1 "ModelParam_GPSLatLong:"; sfcnParam2 "ModelParam_GlobalNoiseGainSwitch:"; sfcnParam3 "ModelParam_envAltitude:"
      mask help: Simulink:masks:GenSFuncDesc_MD
      mask init: same as Exp2_ControlSystemDemo/Quadcopter Dynamics/Battery Model/Battery Model_sfcn
      settings: SFcnIsStateOwnerBlock=on
      settings: CopyFcn=|
      | if ~strcmp(get_param(gcb,'Linkstatus'),'none') && ...
      | ~strcmp(get_param(gcb,'Linkstatus'),'implicit')
      |   set_param(gcb,'LinkStatus','none');
      | end
      mask Help: eval('feval(''rtwprivate'',''rtwhelpview'',''rtw_sfcn_block'')');
      mask Display:
      | port_label('input',1,'PosGPS');
      | port_label('input',2,'gravity');
      | port_label('input',3,'TempC');
      | port_label('input',4,'AirPressure');
      | port_label('input',5,'Rho');
      | port_label('input',6,'Windb');
      | port_label('input',7,'Wind');
      | port_label('input',8,'MotorRads');
      | port_label('input',9,'zt');
      | port_label('input',10,'Fb');
      | port_label('input',11,'Mb');
      | port_label('input',12,'landed');
      | port_label('input',13,'Ve');
      | port_label('input',14,'Xe');
      | port_label('input',15,'Eular(rad)');
      | port_label('input',16,'DCM');
      | port_label('input',17,'Vb');
      | port_label('input',18,'wb');
      | port_label('input',19,'dwb/dt');
      | port_label('input',20,'m');
      | port_label('input',21,'J');
      | port_label('input',22,'dM');
      | port_label('input',23,'PWMOut');
      | port_label('input',24,'cellVol');
      | port_label('input',25,'remCapa');
      | port_label('output',1,'MavLinkSensorData');
      | port_label('output',2,'MavLinkStateQuatData');
      | port_label('output',3,'MavLinkGPSData');
      | port_label('output',4,'HILGPS');
      | port_label('output',5,'MagDec');
      | port_label('output',6,'SysTime');
      | port_label('output',7,'VelE');
      | port_label('output',8,'PosE');
      | port_label('output',9,'AngEuler');
      | port_label('output',10,'AngQuatern');
      | port_label('output',11,'PosGPSb');
      | port_label('output',12,'RateB');
      | port_label('output',13,'AccB');
      | port_label('output',14,'FailInfo');
      | port_label('output',15,'landedb');
      | port_label('output',16,'BattCellVoltage');
      | port_label('output',17,'BattRemCapacity');
      | port_label('output',18,'MotorRPMS');
      | port_label('output',19,'wind');
  __InputSSForSFun__ : Subsystem
  __OutputSSForSFun__ : Subsystem
  MavLinkSensorData : Outport  OutDataTypeStr=Bus: MavLinkSensor  SampleTime=[-1 0]  BusOutputAsStruct=on
  MavLinkStateQuatData : Outport  Port=2  OutDataTypeStr=Bus: MavLinkStateQuat  SampleTime=[-1 0]  BusOutputAsStruct=on
  MavLinkGPSData : Outport  Port=3  OutDataTypeStr=Bus: MavLinkGPS  SampleTime=[-1 0]  BusOutputAsStruct=on
  HILGPS : Outport  Port=4  OutDataTypeStr=Bus: HILGPS  SampleTime=[-1 0]  BusOutputAsStruct=on
  MagDec : Outport  Port=5
  SysTime : Outport  Port=6
  VelE : Outport  Port=7
  PosE : Outport  Port=8
  AngEuler : Outport  Port=9
  AngQuatern : Outport  Port=10
  PosGPS : Outport  Port=11
  RateB : Outport  Port=12
  AccB : Outport  Port=13
  FailInfo : Outport  Port=14
  landed : Outport  Port=15
  BattCellVoltage : Outport  Port=16
  BattRemCapacity : Outport  Port=17
  MotorRPMS : Outport  Port=18
  wind : Outport  Port=19
  wires:
  Environment Model Bus/1 -> __InputSSForSFun__/1(Environment Model Bus)
  MotorRads/1 -> __InputSSForSFun__/2(MotorRads)
  zt/1 -> __InputSSForSFun__/3(zt)
  Force and Moment Model Bus/1 -> __InputSSForSFun__/4(Force and Moment Model Bus)
  6DOF Bus/1 -> __InputSSForSFun__/5(6DOF Bus)
  Fail Model Bus/1 -> __InputSSForSFun__/6(Fail Model Bus)
  Battery Model Bus/1 -> __InputSSForSFun__/7(Battery Model Bus)
  __InputSSForSFun__/1(__UniqueOutportName__1__) -> OutputPort_sfcn/1
  __InputSSForSFun__/2(__UniqueOutportName__2__) -> OutputPort_sfcn/2
  __InputSSForSFun__/3(__UniqueOutportName__3__) -> OutputPort_sfcn/3
  __InputSSForSFun__/4(__UniqueOutportName__4__) -> OutputPort_sfcn/4
  __InputSSForSFun__/5(__UniqueOutportName__5__) -> OutputPort_sfcn/5
  __InputSSForSFun__/6(__UniqueOutportName__6__) -> OutputPort_sfcn/6
  __InputSSForSFun__/7(__UniqueOutportName__7__) -> OutputPort_sfcn/7
  __InputSSForSFun__/8(__UniqueOutportName__8__) -> OutputPort_sfcn/8
  __InputSSForSFun__/9(__UniqueOutportName__9__) -> OutputPort_sfcn/9
  __InputSSForSFun__/10(__UniqueOutportName__10__) -> OutputPort_sfcn/10
  __InputSSForSFun__/11(__UniqueOutportName__11__) -> OutputPort_sfcn/11
  __InputSSForSFun__/12(__UniqueOutportName__12__) -> OutputPort_sfcn/12
  __InputSSForSFun__/13(__UniqueOutportName__13__) -> OutputPort_sfcn/13
  __InputSSForSFun__/14(__UniqueOutportName__14__) -> OutputPort_sfcn/14
  __InputSSForSFun__/15(__UniqueOutportName__15__) -> OutputPort_sfcn/15
  __InputSSForSFun__/16(__UniqueOutportName__16__) -> OutputPort_sfcn/16
  __InputSSForSFun__/17(__UniqueOutportName__17__) -> OutputPort_sfcn/17
  __InputSSForSFun__/18(__UniqueOutportName__18__) -> OutputPort_sfcn/18
  __InputSSForSFun__/19(__UniqueOutportName__19__) -> OutputPort_sfcn/19
  __InputSSForSFun__/20(__UniqueOutportName__20__) -> OutputPort_sfcn/20
  __InputSSForSFun__/21(__UniqueOutportName__21__) -> OutputPort_sfcn/21
  __InputSSForSFun__/22(__UniqueOutportName__22__) -> OutputPort_sfcn/22
  __InputSSForSFun__/23(__UniqueOutportName__23__) -> OutputPort_sfcn/23
  __InputSSForSFun__/24(__UniqueOutportName__24__) -> OutputPort_sfcn/24
  __InputSSForSFun__/25(__UniqueOutportName__25__) -> OutputPort_sfcn/25
  OutputPort_sfcn/1 -> __OutputSSForSFun__/1(__UniqueInportName__1__)
  OutputPort_sfcn/2 -> __OutputSSForSFun__/2(__UniqueInportName__2__)
  OutputPort_sfcn/3 -> __OutputSSForSFun__/3(__UniqueInportName__3__)
  OutputPort_sfcn/4 -> __OutputSSForSFun__/4(__UniqueInportName__4__)
  OutputPort_sfcn/5 -> __OutputSSForSFun__/5(__UniqueInportName__5__)
  OutputPort_sfcn/6 -> __OutputSSForSFun__/6(__UniqueInportName__6__)
  OutputPort_sfcn/7 -> __OutputSSForSFun__/7(__UniqueInportName__7__)
  OutputPort_sfcn/8 -> __OutputSSForSFun__/8(__UniqueInportName__8__)
  OutputPort_sfcn/9 -> __OutputSSForSFun__/9(__UniqueInportName__9__)
  OutputPort_sfcn/10 -> __OutputSSForSFun__/10(__UniqueInportName__10__)
  OutputPort_sfcn/11 -> __OutputSSForSFun__/11(__UniqueInportName__11__)
  OutputPort_sfcn/12 -> __OutputSSForSFun__/12(__UniqueInportName__12__)
  OutputPort_sfcn/13 -> __OutputSSForSFun__/13(__UniqueInportName__13__)
  OutputPort_sfcn/14 -> __OutputSSForSFun__/14(__UniqueInportName__14__)
  OutputPort_sfcn/15 -> __OutputSSForSFun__/15(__UniqueInportName__15__)
  OutputPort_sfcn/16 -> __OutputSSForSFun__/16(__UniqueInportName__16__)
  OutputPort_sfcn/17 -> __OutputSSForSFun__/17(__UniqueInportName__17__)
  OutputPort_sfcn/18 -> __OutputSSForSFun__/18(__UniqueInportName__18__)
  OutputPort_sfcn/19 -> __OutputSSForSFun__/19(__UniqueInportName__19__)
  __OutputSSForSFun__/1(MavLinkSensorData) -> MavLinkSensorData/1
  __OutputSSForSFun__/2(MavLinkStateQuatData) -> MavLinkStateQuatData/1
  __OutputSSForSFun__/3(MavLinkGPSData) -> MavLinkGPSData/1
  __OutputSSForSFun__/4(HILGPS) -> HILGPS/1
  __OutputSSForSFun__/5(MagDec) -> MagDec/1
  __OutputSSForSFun__/6(SysTime) -> SysTime/1
  __OutputSSForSFun__/7(VelE) -> VelE/1
  __OutputSSForSFun__/8(PosE) -> PosE/1
  __OutputSSForSFun__/9(AngEuler) -> AngEuler/1
  __OutputSSForSFun__/10(AngQuatern) -> AngQuatern/1
  __OutputSSForSFun__/11(PosGPS) -> PosGPS/1
  __OutputSSForSFun__/12(RateB) -> RateB/1
  __OutputSSForSFun__/13(AccB) -> AccB/1
  __OutputSSForSFun__/14(FailInfo) -> FailInfo/1
  __OutputSSForSFun__/15(landed) -> landed/1
  __OutputSSForSFun__/16(BattCellVoltage) -> BattCellVoltage/1
  __OutputSSForSFun__/17(BattRemCapacity) -> BattRemCapacity/1
  __OutputSSForSFun__/18(MotorRPMS) -> MotorRPMS/1
  __OutputSSForSFun__/19(wind) -> wind/1

== system Exp2_ControlSystemDemo/Quadcopter Dynamics/Separation of float Data1 ==
  note: 小数部分
  float_Data : Inport
  Add2 : Sum  Inputs=+-
  Integer Uint : Constant  Value=IntUint
  Math Function1 : Math  Operator=mod  SaturateOnIntegerOverflow=on
  Integer_Part : Outport
  decimalt_Part : Outport  Port=2
  wires:
  Math Function1/1 -> decimalt_Part/1, Add2/2
  Integer Uint/1 -> Math Function1/2
  Add2/1 -> Integer_Part/1
  float_Data/1 -> Math Function1/1, Add2/1

== system Exp2_ControlSystemDemo/Subsystem/ARMINGControl ==
  In1 : Inport
  Compare To Constant3 : simulink/Logic and Bit Operations/Compare To Constant  relop=>=  const=uint16(1500)  OutDataTypeStr=boolean
  Out1 : Outport
  wires:
  Compare To Constant3/1 -> Out1/1
  In1/1 -> Compare To Constant3/1
